simulink model "MSE452_Lab3_PMSM_ForStudent"  (R2023a)
settings: Solver=ode45  StartTime=0.0  StopTime=0.3  MaxStep=1e-5  RelTol=1e-3  EnableMultiTasking=on
InitFcn:
  | Idc=0;
  | Vabc=0;
  | Iw=0;
values from neighbouring files (symbols this model uses):
  Flux = 0.7213*BaseFlux    [MSE452_Lab3_parameters.m]
  Ld = 0.7029*Lb    [MSE452_Lab3_parameters.m]
  Lq = 0.7029*Lb    [MSE452_Lab3_parameters.m]
  OMEGAb_r = OMEGAb/Ppairs    (= 41.885284054)    [MSE452_Lab3_parameters.m]
  Ppairs = 8    [MSE452_Lab3_parameters.m]
  R = Pb/(3*(Ib^2))    [MSE452_Lab3_parameters.m]
  Rs = 0.00517*Zb    [MSE452_Lab3_parameters.m]
  Tm = 58.4585e3    (= 58458.5)    [MSE452_Lab3_parameters.m]
undefined symbols (not defined in the file or in its folder): Ts
libraries: spspowerguiLib x1
settings Model: Creator=Administrator  LastModifiedBy=auamai
settings SolverCC: ZeroCrossControl=DisableAll  AlgebraicLoopSolver=TrustRegion
settings DataIOCC: LimitDataPoints=on  SaveFormat=Array  SignalLoggingSaveFormat=ModelDataLogs  ReturnWorkspaceOutputs=off
settings OptimizationCC: BlockReduction=off  DefaultParameterBehavior=Inlined  BufferReuse=off  ExpressionDepthLimit=2147483647  InitFltsAndDblsToZero=on  LifeSpan=inf
settings DebuggingCC: SaveWithParameterizedLinksMsg=none  UnderspecifiedInitializationDetection=Classic  MergeDetectMultiDrivingBlocksExec=none  SignalResolutionControl=TryResolveAllWithWarning  SolverPrmCheckMsg=warning  MultiTaskDSMMsg=warning  MultiTaskCondExecSysMsg=none  FcnCallInpInsideContextMsg=warning  UnconnectedInputMsg=warning  UnconnectedOutputMsg=warning  UnconnectedLineMsg=warning  StateNameClashWarn=warning  SFUnexpectedBacktrackingDiag=warning  SFNoUnconditionalDefaultTransitionDiag=warning  SFExecutionAtInitializationDiag=none  ArithmeticOperatorsInVariantConditions=warning
settings HardwareCC: ProdBitPerPointer=32  ProdBitPerSizeT=32  ProdBitPerPtrDiffT=32  ProdLargestAtomicFloat=None  ProdIntDivRoundTo=Undefined  ProdEndianess=Unspecified  ProdWordSize=32  ProdHWDeviceType=32-bit Generic
settings ModelReferenceCC: PropagateSignalLabelsOutOfModel=off
settings SFSimCC: SimUseLocalCustomCode=off  CustomCodeUndefinedFunction=UseInterfaceOnly
settings RTWCC: RTWUseLocalCustomCode=off
settings CodeAppCC: StateflowObjectComments=on
settings GRTTargetCC: TargetFcnLib=ansi_tfl_tmw.mat  TargetLangStandard=C89/C90 (ANSI)  CombineOutputUpdateFcns=off  GRTInterface=on
settings ConfigComp: CovMetricSettings=dw  CovSaveCumulativeToWorkspaceVar=on  CovSaveSingleToWorkspaceVar=on  CovExternalEMLEnable=off

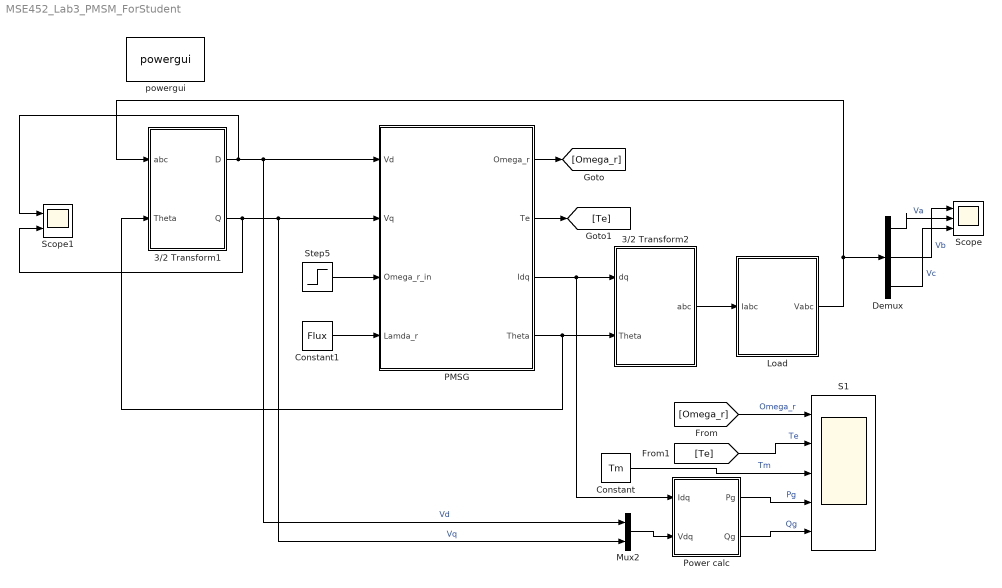
== system MSE452_Lab3_PMSM_ForStudent ==
  3/2 Transform1 : Subsystem
  3/2 Transform2 : Subsystem
  Constant : Constant  Value=Tm
  Constant1 : Constant  Value=Flux
  Demux : Demux  Outputs=3
  Load : Subsystem
  Mux2 : Mux  Inputs=2
  PMSG : Subsystem
  Power calc : Subsystem
  S1 : Scope  NumInputPorts=5
  Scope : Scope  NumInputPorts=3
  Scope1 : Scope  NumInputPorts=2
  Step5 : Step  Time=0  After=0.8*OMEGAb_r  SampleTime=0
  powergui : spspowerguiLib/powergui  SimulationMode=Continuous  SampleTime=Ts  frequency=60  Iterations=50  frequencyindice=1  Pbase=100e6  ErrMax=1e-4  UnitsV=kV  UnitsW=MW  buscounter=0  FunctionMessages=off  echomessages=off  EnableUseOfTLC=off  CurrentSourceSwitches=on  DisableSnubberDevices=off  DisableRonSwitches=off  DisableVfSwitches=off  DisplayEquations=off  AutomaticDiscreteSolvers=off  SolverType=Tustin  Interpol=off  ExternalGateDelay=off  methode=off  Ts=0  x0status=blocks  SPID=off  SwTol=0  HookPort=off  NonlinearTolerance=1e-4  nMaxIteration=100  ContinueOnMaxIteration=off  RestoreLinks=warning  ResistiveCurrentMeasurement=off  Frange=[0:2:500]  Ylog=off  Xlog=on  ShowGrid=off  save=off  variable=ZData  structure=GridVIWave  ZoomFFT=off  StartTime=2  cycles=12  DisplayStyle=1  fundamental=60  FreqAxis=on  MaxFrequency=60*15  frequencyindicesteady=1  RmsSteady=1  display=off
  wires:
  PMSG/3(Idq) -> 3/2 Transform2/1(dq), Power calc/1(Idq)
  3/2 Transform1/2(Q) -> Scope1/2, PMSG/2(Vq), Mux2/2  "Vq"
  3/2 Transform1/1(D) -> Scope1/1, PMSG/1(Vd), Mux2/1  "Vd"
  PMSG/1(Omega_r) -> [Omega_r]
  PMSG/2(Te) -> [Te]
  Step5/1 -> PMSG/3(Omega_r_in)
  PMSG/4(Theta) -> 3/2 Transform2/2(Theta), 3/2 Transform1/2(Theta)
  Mux2/1 -> Power calc/2(Vdq)
  Constant1/1 -> PMSG/4(Lamda_r)
  3/2 Transform2/1(abc) -> Load/1(Iabc)
  Load/1(Vabc) -> 3/2 Transform1/1(abc), Demux/1
  Power calc/2(Qg) -> S1/5  "Qg"
  Power calc/1(Pg) -> S1/4  "Pg"
  [Omega_r] -> S1/1  "Omega_r"
  [Te] -> S1/2  "Te"
  Demux/1 -> Scope/2  "Va"
  Demux/2 -> Scope/1  "Vb"
  Demux/3 -> Scope/3  "Vc"
  Constant/1 -> S1/3  "Tm"

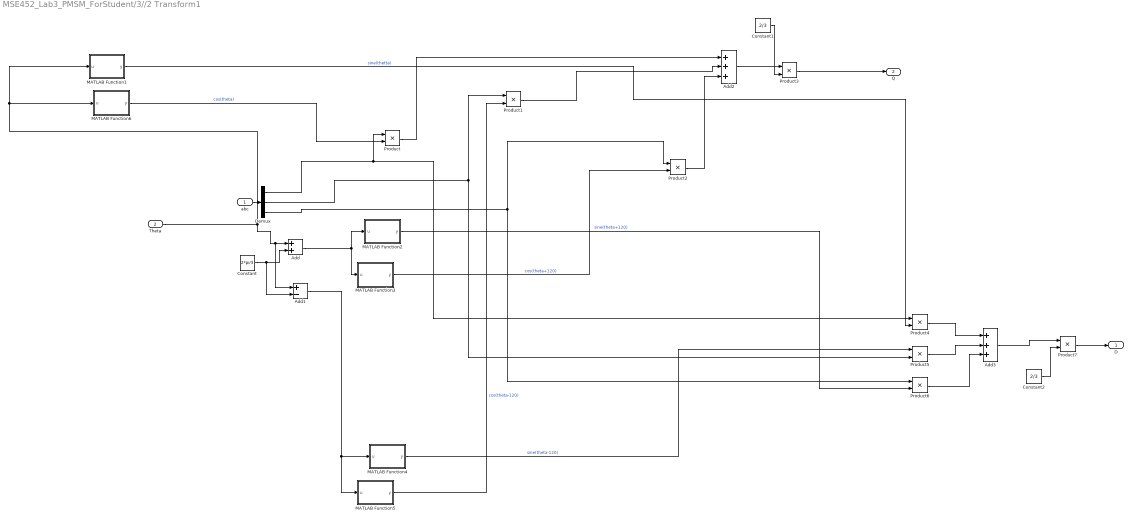
== system MSE452_Lab3_PMSM_ForStudent/3//2 Transform1 ==
  abc : Inport
  Theta : Inport  Port=2
  Add : Sum
  Add1 : Sum  Inputs=+-
  Add2 : Sum  Inputs=+++
  Add3 : Sum  Inputs=+++
  Constant : Constant  Value=2*pi/3
  Constant1 : Constant  Value=2/3
  Constant2 : Constant  Value=2/3
  Demux : Demux  Outputs=3
  MATLAB Function1 : MATLAB Function  TreatAsAtomicUnit=on
  MATLAB Function2 : MATLAB Function  TreatAsAtomicUnit=on
  MATLAB Function3 : MATLAB Function  TreatAsAtomicUnit=on
  MATLAB Function4 : MATLAB Function  TreatAsAtomicUnit=on
  MATLAB Function5 : MATLAB Function  TreatAsAtomicUnit=on
  MATLAB Function6 : MATLAB Function  TreatAsAtomicUnit=on
  Product{,1..7} (8 alike) : Product
  D : Outport
  Q : Outport  Port=2
  wires:
  abc/1 -> Demux/1
  Demux/1 -> Product4/1, Product/1
  Demux/2 -> Product5/2, Product1/1
  Demux/3 -> Product6/1, Product2/1
  Theta/1 -> Add1/1, Add/1, MATLAB Function6/1(u), MATLAB Function1/1(u)
  Constant/1 -> Add1/2, Add/2
  MATLAB Function2/1(y) -> Product6/2  "sine(theta+120)"
  Add/1 -> MATLAB Function3/1(u), MATLAB Function2/1(u)
  MATLAB Function3/1(y) -> Product2/2  "cos(theta+120)"
  MATLAB Function4/1(y) -> Product5/1  "sine(theta-120)"
  Add1/1 -> MATLAB Function5/1(u), MATLAB Function4/1(u)
  MATLAB Function5/1(y) -> Product1/2  "cos(theta-120)"
  MATLAB Function1/1(y) -> Product4/2  "sine(thetta)"
  MATLAB Function6/1(y) -> Product/2  "cos(theta)"
  Product/1 -> Add2/1
  Product1/1 -> Add2/2
  Product2/1 -> Add2/3
  Add2/1 -> Product3/1
  Constant1/1 -> Product3/2
  Product3/1 -> Q/1
  Product4/1 -> Add3/1
  Product5/1 -> Add3/2
  Product6/1 -> Add3/3
  Add3/1 -> Product7/1
  Constant2/1 -> Product7/2
  Product7/1 -> D/1

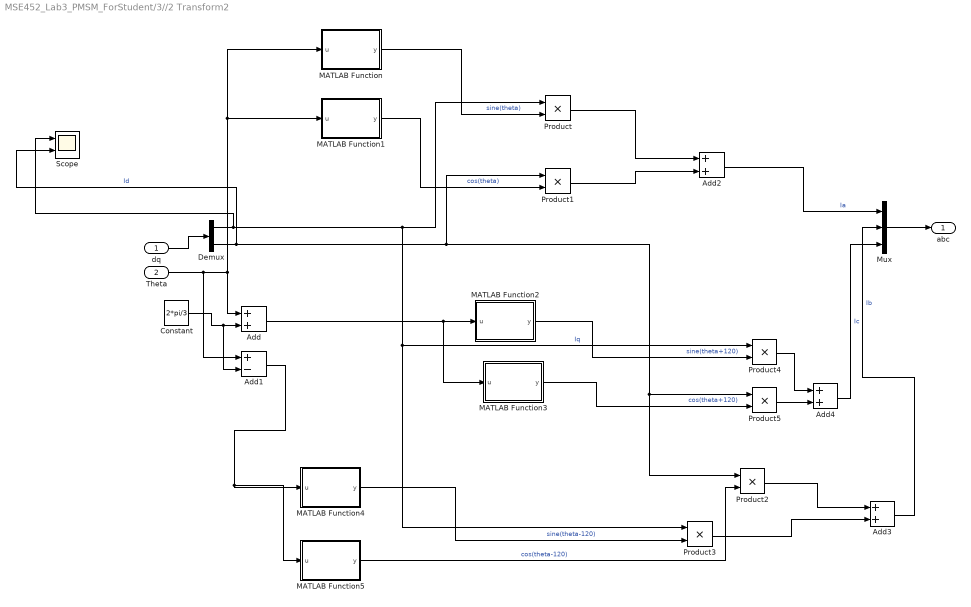
== system MSE452_Lab3_PMSM_ForStudent/3//2 Transform2 ==
  dq : Inport
  Theta : Inport  Port=2
  Add{,2..4} (4 alike) : Sum
  Add1 : Sum  Inputs=+-
  Constant : Constant  Value=2*pi/3
  Demux : Demux  Outputs=2
  MATLAB Function : MATLAB Function  TreatAsAtomicUnit=on
  MATLAB Function1 : MATLAB Function  TreatAsAtomicUnit=on
  MATLAB Function2 : MATLAB Function  TreatAsAtomicUnit=on
  MATLAB Function3 : MATLAB Function  TreatAsAtomicUnit=on
  MATLAB Function4 : MATLAB Function  TreatAsAtomicUnit=on
  MATLAB Function5 : MATLAB Function  TreatAsAtomicUnit=on
  Mux : Mux  Inputs=3
  Product{,1..5} (6 alike) : Product
  Scope : Scope  NumInputPorts=2
  abc : Outport
  wires:
  dq/1 -> Demux/1
  Demux/2 -> Scope/2, Product5/1, Product2/1, Product1/1  "Id"
  Constant/1 -> Add1/2, Add/2
  Theta/1 -> Add1/1, MATLAB Function1/1(u), MATLAB Function/1(u), Add/1
  MATLAB Function/1(y) -> Product/2  "sine(theta)"
  MATLAB Function1/1(y) -> Product1/2  "cos(theta)"
  Demux/1 -> Scope/1, Product4/1, Product3/1, Product/1  "Iq"
  Product/1 -> Add2/1
  Product1/1 -> Add2/2
  Add2/1 -> Mux/1  "Ia"
  Mux/1 -> abc/1
  Add/1 -> MATLAB Function3/1(u), MATLAB Function2/1(u)
  MATLAB Function2/1(y) -> Product4/2  "sine(theta+120)"
  MATLAB Function3/1(y) -> Product5/2  "cos(theta+120)"
  Add1/1 -> MATLAB Function5/1(u), MATLAB Function4/1(u)
  MATLAB Function4/1(y) -> Product3/2  "sine(theta-120)"
  MATLAB Function5/1(y) -> Product2/2  "cos(theta-120)"
  Product2/1 -> Add3/1
  Product3/1 -> Add3/2
  Add3/1 -> Mux/2  "Ib"
  Product4/1 -> Add4/1
  Product5/1 -> Add4/2
  Add4/1 -> Mux/3  "Ic"

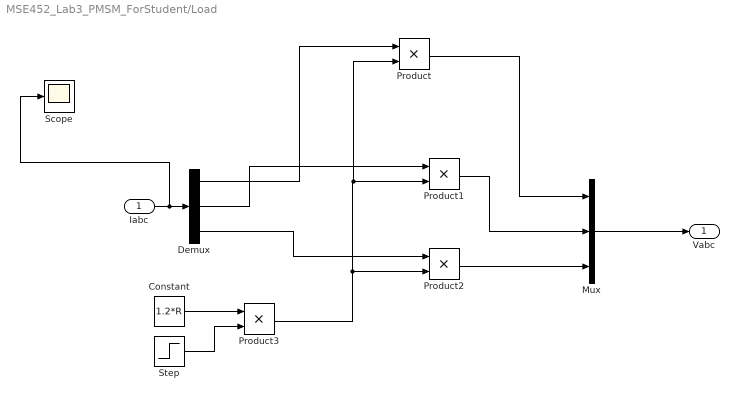
== system MSE452_Lab3_PMSM_ForStudent/Load ==
  Iabc : Inport
  Constant : Constant  Value=1.2*R
  Demux : Demux  Outputs=3
  Mux : Mux  Inputs=3
  Product{,1..3} (4 alike) : Product
  Scope : Scope
  Step : Step  Time=0.1  Before=1  After=1/2  SampleTime=0
  Vabc : Outport
  wires:
  Iabc/1 -> Scope/1, Demux/1
  Demux/1 -> Product/1
  Product/1 -> Mux/1
  Demux/2 -> Product1/1
  Demux/3 -> Product2/1
  Product1/1 -> Mux/2
  Product2/1 -> Mux/3
  Mux/1 -> Vabc/1
  Product3/1 -> Product/2, Product1/2, Product2/2
  Constant/1 -> Product3/1
  Step/1 -> Product3/2

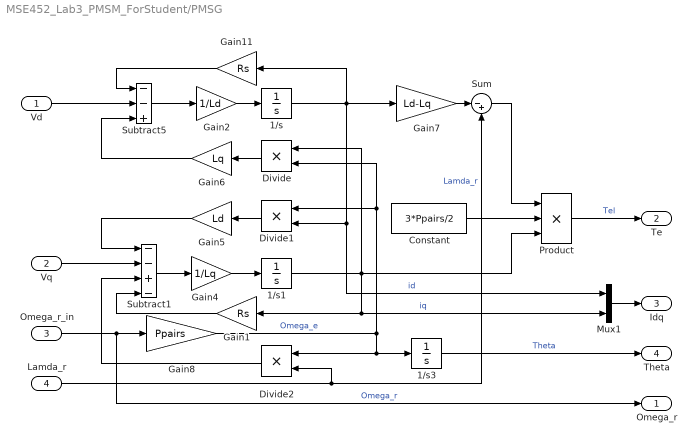
== system MSE452_Lab3_PMSM_ForStudent/PMSG ==
  Vd : Inport
  Vq : Inport  Port=2
  Omega_r_in : Inport  Port=3
  Lamda_r : Inport  Port=4
  1/s : Integrator
  1/s1 : Integrator
  1/s3 : Integrator
  Constant : Constant  Value=3*Ppairs/2
  Divide : Product  Inputs=**
  Divide1 : Product  Inputs=**
  Divide2 : Product  Inputs=**
  Gain1 : Gain  Gain=Rs
  Gain11 : Gain  Gain=Rs
  Gain2 : Gain  Gain=1/Ld
  Gain4 : Gain  Gain=1/Lq
  Gain5 : Gain  Gain=Ld
  Gain6 : Gain  Gain=Lq
  Gain7 : Gain  Gain=Ld-Lq
  Gain8 : Gain  Gain=Ppairs
  Mux1 : Mux  Inputs=2
  Product : Product  Inputs=3  RndMeth=Zero
  Subtract1 : Sum  Inputs=--+-
  Subtract5 : Sum  Inputs=--+
  Sum : Sum  Inputs=|-+
  Omega_r : Outport
  Te : Outport  Port=2
  Idq : Outport  Port=3
  Theta : Outport  Port=4
  wires:
  Divide2/1 -> Subtract1/3
  Product/1 -> Te/1  "Tel"
  Constant/1 -> Product/2
  Sum/1 -> Product/1
  Gain7/1 -> Sum/1
  Gain5/1 -> Subtract1/1
  Gain6/1 -> Subtract5/3
  Divide1/1 -> Gain5/1
  Divide/1 -> Gain6/1
  1/s1/1 -> Divide/1, Product/3, Mux1/2, Gain1/1  "iq"
  Gain4/1 -> 1/s1/1
  Subtract1/1 -> Gain4/1
  1/s/1 -> Divide1/2, Mux1/1, Gain7/1, Gain11/1  "id"
  Gain2/1 -> 1/s/1
  Subtract5/1 -> Gain2/1
  Vd/1 -> Subtract5/2
  Vq/1 -> Subtract1/2
  Mux1/1 -> Idq/1
  Gain11/1 -> Subtract5/1
  Lamda_r/1 -> Divide2/2, Sum/2  "Lamda_r"
  Omega_r_in/1 -> Gain8/1, Omega_r/1  "Omega_r"
  1/s3/1 -> Theta/1  "Theta"
  Gain1/1 -> Subtract1/4
  Gain8/1 -> Divide1/1, Divide/2, Divide2/1, 1/s3/1  "Omega_e"

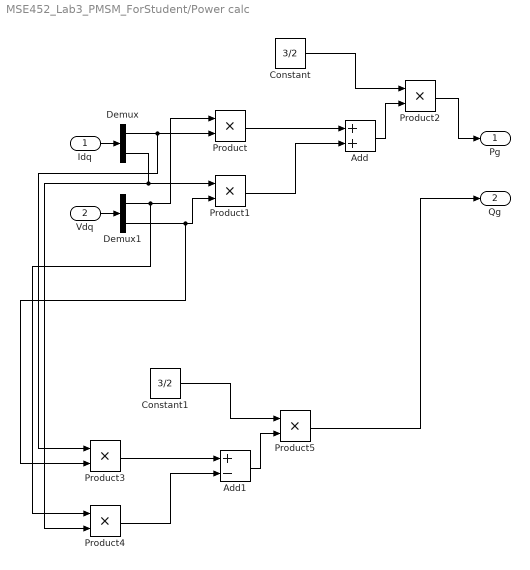
== system MSE452_Lab3_PMSM_ForStudent/Power calc ==
  Idq : Inport
  Vdq : Inport  Port=2
  Add : Sum
  Add1 : Sum  Inputs=+-
  Constant : Constant  Value=3/2
  Constant1 : Constant  Value=3/2
  Demux : Demux  Outputs=2
  Demux1 : Demux  Outputs=2
  Product{,1..5} (6 alike) : Product
  Pg : Outport
  Qg : Outport  Port=2
  wires:
  Vdq/1 -> Demux1/1
  Idq/1 -> Demux/1
  Demux1/1 -> Product4/1, Product/1
  Demux/1 -> Product3/1, Product/2
  Product/1 -> Add/1
  Demux1/2 -> Product3/2, Product1/2
  Demux/2 -> Product1/1, Product4/2
  Product1/1 -> Add/2
  Add/1 -> Product2/2
  Constant/1 -> Product2/1
  Product2/1 -> Pg/1
  Constant1/1 -> Product5/1
  Add1/1 -> Product5/2
  Product4/1 -> Add1/2
  Product3/1 -> Add1/1
  Product5/1 -> Qg/1

== matlab function MSE452_Lab3_PMSM_ForStudent/3//2 Transform2/MATLAB Function ==
  data: u input; y output
function y = fcn(u)

y = sin(u);

== matlab function MSE452_Lab3_PMSM_ForStudent/3//2 Transform2/MATLAB Function2 ==
  data: u input; y output
function y = fcn(u)

y = sin(u);

== matlab function MSE452_Lab3_PMSM_ForStudent/3//2 Transform2/MATLAB Function3 ==
  data: u input; y output
function y = fcn(u)

y = cos(u);

== matlab function MSE452_Lab3_PMSM_ForStudent/3//2 Transform2/MATLAB Function4 ==
  data: u input; y output
function y = fcn(u)

y = sin(u);

== matlab function MSE452_Lab3_PMSM_ForStudent/3//2 Transform2/MATLAB Function5 ==
  data: u input; y output
function y = fcn(u)

y = cos(u);

== matlab function MSE452_Lab3_PMSM_ForStudent/3//2 Transform1/MATLAB Function2 ==
  data: u input; y output
function y = fcn(u)

y = sin(u);

== matlab function MSE452_Lab3_PMSM_ForStudent/3//2 Transform1/MATLAB Function3 ==
  data: u input; y output
function y = fcn(u)

y = cos(u);

== matlab function MSE452_Lab3_PMSM_ForStudent/3//2 Transform1/MATLAB Function4 ==
  data: u input; y output
function y = fcn(u)

y = sin(u);

== matlab function MSE452_Lab3_PMSM_ForStudent/3//2 Transform2/MATLAB Function1 ==
  data: u input; y output
function y = fcn(u)

y = cos(u);

== matlab function MSE452_Lab3_PMSM_ForStudent/3//2 Transform1/MATLAB Function5 ==
  data: u input; y output
function y = fcn(u)

y = cos(u);

== matlab function MSE452_Lab3_PMSM_ForStudent/3//2 Transform1/MATLAB Function1 ==
  data: u input; y output
function y = fcn(u)

y = sin(u);

== matlab function MSE452_Lab3_PMSM_ForStudent/3//2 Transform1/MATLAB Function6 ==
  data: u input; y output
function y = fcn(u)

y = cos(u);
